simulink model "KalmanMPC2024a"  (R2024a)
settings: Solver=VariableStepAuto  StartTime=0.0  StopTime=10  RelTol=1e-3
values from neighbouring files (symbols this model uses):
  B_noise = [Bd ones(size(Bd,1),1)]    [scriptpoint7.m]
  D_noise = [Dd zeros(size(Dd,1),1)]    [scriptpoint7.m]
  N = 5    [project_script.m]    (also in scriptpoint7.m)
  NK = 0    [scriptpoint7.m]
  Qd = 1*eye(2)    [project_script.m]    (also in scriptpoint7.m = 1000*eye(2))
  Rd = 1*eye(2)    [project_script.m]    (also in scriptpoint7.m)
  RK = 1*eye(2)    [scriptpoint7.m]
  Ts = 1/8000    (= 0.000125)    [project_script.m]    (also in scriptpoint7.m)
  u_bar_d = Bd\ (eye(size(Ad))-Ad)*xref    [project_script.m]    (also in scriptpoint7.m)
  u_sat_max = [u1_max; u2_max]    [project_script.m]    (also in scriptpoint7.m)
  u_sat_min = [u1_min; u2_min]    [project_script.m]    (also in scriptpoint7.m)
  x0 = [x0_1;x0_2]    [project_script.m]    (also in scriptpoint7.m)
  x0K = 1.5*x0    [scriptpoint7.m]
  x_sat_max = [x1_max; x2_max]    [project_script.m]    (also in scriptpoint7.m)
  x_sat_min = [x1_min; x2_min]    [project_script.m]    (also in scriptpoint7.m)
  xref = [6.9; 8.9]    [project_script.m]    (also in scriptpoint7.m)
undefined symbols (not defined in the file or in its folder): Ad, Bd, Cd, Dd, Discrete, mympc, Sd, Time
libraries: simulink x2, ctrlSharedLib x1
settings Model: Creator=Utente  LastModifiedBy=papidrago

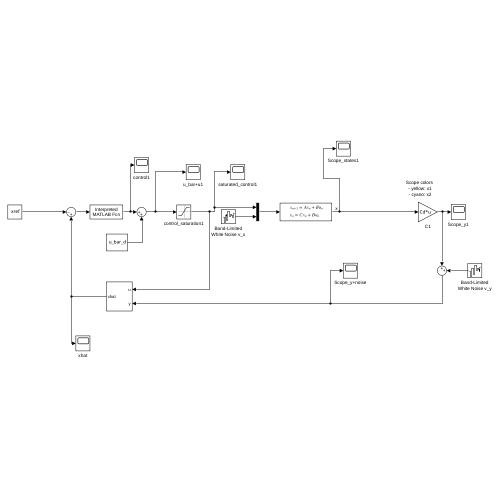
[thumbnail: Simulink's stored preview of the top-level diagram]
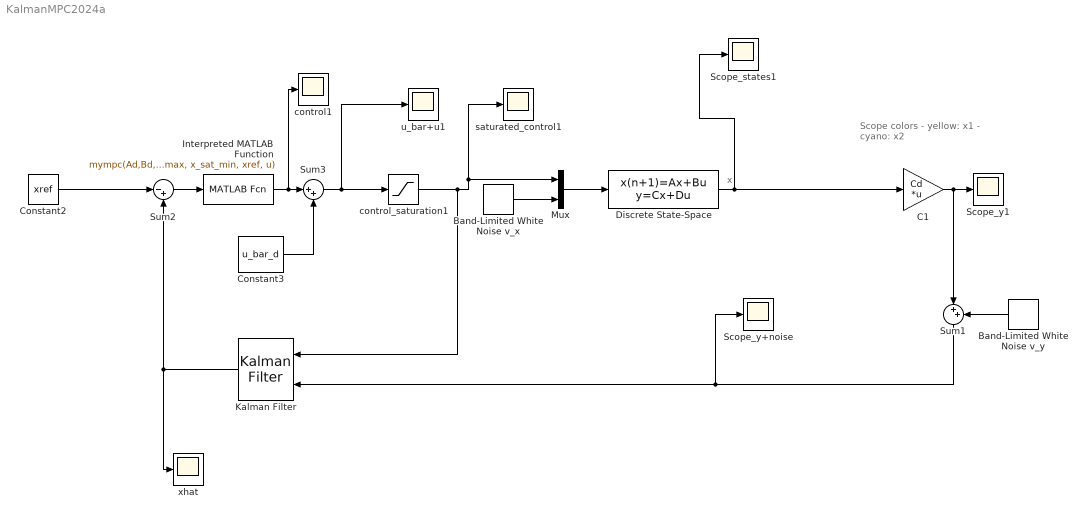
== system KalmanMPC2024a ==
  note: x
  note: Scope colors
      | - yellow: x1
      | - cyano: x2
  Band-Limited White Noise v_x : simulink/Sources/Band-Limited White Noise  Cov=power_vx  Ts=Ts  seed=[123]
  Band-Limited White Noise v_y : simulink/Sources/Band-Limited White Noise  Cov=power_vy  Ts=Ts  seed=[456]
  C1 : Gain  Gain=Cd  Multiplication=Matrix(K*u)
  Constant2 : Constant  Value=xref  SampleTime=Ts
  Constant3 : Constant  Value=u_bar_d  SampleTime=Ts
  Discrete State-Space : DiscreteStateSpace  A=Ad  B=B_noise  C=Cd  D=D_noise  InitialCondition=x0  SampleTime=Ts
  Interpreted MATLAB Function : MATLABFcn  MATLABFcn=mympc(Ad,Bd,Qd,Rd,Sd,N,u_sat_min,u_sat_max,u_bar_d, x_sat_max, x_sat_min, xref, u)
  Kalman Filter : ctrlSharedLib/Kalman Filter  TimeDomain=Discrete-Time  UseCurrentEstimator=on  ModelSource=Individual A, B, C, D matrices  ModelSourceVariable=ss(0.95,1,1,0,1)  A=Ad  B=Bd  C=Cd  D=Dd  NumberOfStates=1  NumberOfInputs=1  NumberOfOutputs=1  InitialEstimateSource=Dialog  X0=x0K  P0=10  UseK=off  UseGH=off  NumberOfProcessNoiseInputs=1  G=1  TimeInvariantG=on  H=0  TimeInvariantH=on  Q=QK  TimeInvariantQ=on  R=RK  TimeInvariantR=on  N=NK  TimeInvariantN=on  AddInputPort=on  AddEnablePort=off  OutputEstimatedY=off  OutputP=off  Ts=-1
  Mux : Mux  Inputs=2
  Scope_states1 : Scope
  Scope_y+noise : Scope
  Scope_y1 : Scope
  Sum1 : Sum  Inputs=|++
  Sum2 : Sum  Inputs=|-+
  Sum3 : Sum  Inputs=|++
  control1 : Scope
  control_saturation1 : Saturate  UpperLimit=u_sat_max  LowerLimit=u_sat_min
  saturated_control1 : Scope
  u_bar+u1 : Scope
  xhat : Scope
  wires:
  Discrete State-Space/1 -> C1/1, Scope_states1/1
  Constant3/1 -> Sum3/2
  C1/1 -> Scope_y1/1, Sum1/1
  Interpreted MATLAB Function/1 -> control1/1, Sum3/1
  Constant2/1 -> Sum2/1
  Sum3/1 -> control_saturation1/1, u_bar+u1/1
  Sum2/1 -> Interpreted MATLAB Function/1
  Kalman Filter/1 -> xhat/1, Sum2/2
  control_saturation1/1 -> Kalman Filter/1, Mux/1, saturated_control1/1
  Band-Limited White Noise v_y/1 -> Sum1/2
  Sum1/1 -> Kalman Filter/2, Scope_y+noise/1
  Band-Limited White Noise v_x/1 -> Mux/2
  Mux/1 -> Discrete State-Space/1
